simulink model "Control_sk_R3GDL"  (R2017b)
settings: Solver=ode45  StartTime=0.0  StopTime=12  MaxStep=1e-3  RelTol=1e-3  EnableMultiTasking=on
InitFcn:
  | Ts=1e-3;
StartFcn:
  | Ts=1e-3;
undefined symbols (not defined in the file or in its folder): CinematicaDirecta
settings Model: ExtModeTrigMode=oneshot  ExtModeArmWhenConnect=off  Creator=mortega  LastModifiedBy=Raúl
settings DataIOCC: SaveFormat=Array  SignalLoggingSaveFormat=ModelDataLogs
settings OptimizationCC: BlockReduction=off  BooleanDataType=off  ExpressionDepthLimit=2147483647  InitFltsAndDblsToZero=on  LifeSpan=inf
settings DebuggingCC: SaveWithParameterizedLinksMsg=none  UnderspecifiedInitializationDetection=Classic  MergeDetectMultiDrivingBlocksExec=none  SignalResolutionControl=TryResolveAllWithWarning  MultiTaskDSMMsg=warning  MultiTaskCondExecSysMsg=none  FcnCallInpInsideContextMsg=warning  StateNameClashWarn=warning  SFUnexpectedBacktrackingDiag=warning  SFNoUnconditionalDefaultTransitionDiag=warning  SFExecutionAtInitializationDiag=none
settings HardwareCC: ProdBitPerPointer=32  ProdBitPerSizeT=32  ProdBitPerPtrDiffT=32  ProdLargestAtomicFloat=None  ProdIntDivRoundTo=Undefined  ProdEndianess=Unspecified  ProdWordSize=32  ProdHWDeviceType=32-bit Generic  TargetUnknown=on
settings ModelReferenceCC: PropagateSignalLabelsOutOfModel=off
settings CodeAppCC: StateflowObjectComments=on
settings GRTTargetCC: TargetFcnLib=ansi_tfl_tmw.mat  TargetLangStandard=C89/C90 (ANSI)  GeneratePreprocessorConditionals=Disable all  CombineOutputUpdateFcns=off  GRTInterface=on
settings ConfigComp: CovMetricSettings=dw  CovHtmlReporting=on  CovSaveCumulativeToWorkspaceVar=on  CovSaveSingleToWorkspaceVar=on  CovExternalEMLEnable=off  CovSFcnEnable=off

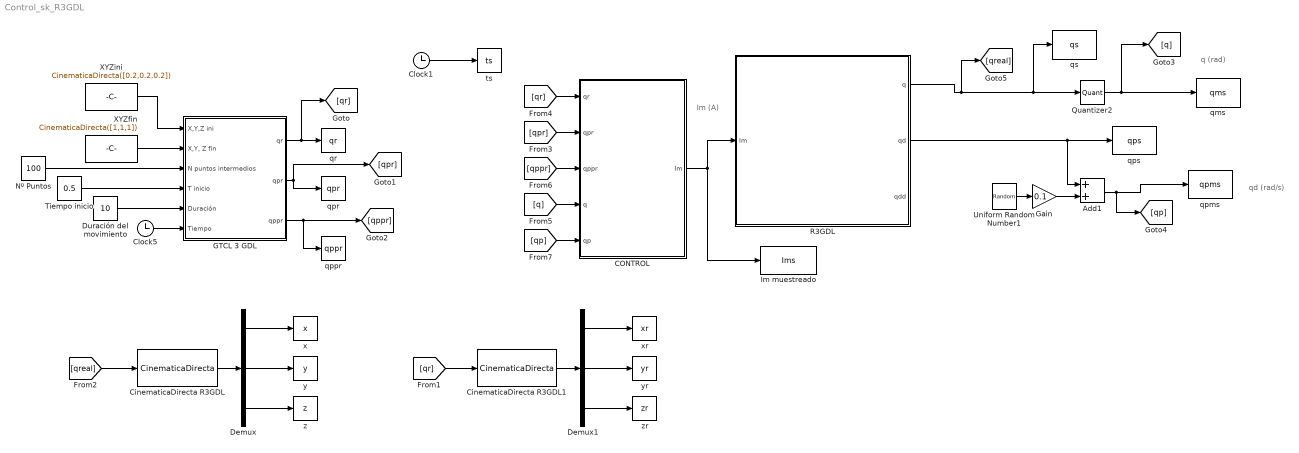
== system Control_sk_R3GDL ==
  note: q (rad)
  note: qd (rad/s)
  note: Im (A)
  Add1 : Sum
  CONTROL : Subsystem
  CinematicaDirecta R3GDL : MATLABFcn  MATLABFcn=CinematicaDirecta
  CinematicaDirecta R3GDL1 : MATLABFcn  MATLABFcn=CinematicaDirecta
  Clock1 : Clock
  Clock5 : Clock
  Demux : Demux  Outputs=3
  Demux1 : Demux  Outputs=3
  Duración del movimiento : Constant  Value=10
  GTCL 3 GDL : Subsystem
  Gain : Gain  Gain=0.1
  Im muestreado : ToWorkspace  VariableName=Ims  SampleTime=1e-3
  Nº Puntos : Constant  Value=100
  Quantizer2 : Quantizer  QuantizationInterval=2*pi/(512*25*100)
  R3GDL : Subsystem  mask(Control y Programación de Robots (4 GIERM)){NGrupo=3, q1_ini=0.2, q2_ini=0.2, q3_ini=0.2, Bl_q1=off, Bl_q2=off, Bl_q3=off, AccionamientoDirecto=on}
      mask prompts: NGrupo "Nº de GRUPO"; q1_ini "q1 inicial  (rad)"; q2_ini "q2 inicial (rad)"; q3_ini "q3_inicial (rad)"; Bl_q1 "Bloqueo q1"; Bl_q2 "Bloqueo q2"; Bl_q3 "Bloqueo q3"; AccionamientoDirecto "Accionamiento directo"
      mask help: Robot de 3 grados de libertad RRR
      mask Display:
      | image(imread('R3GDL_RRR.JPG'));
      | port_label('output', 1, 'q');
      | port_label('output', 2, 'qd');
      | port_label('output', 3, 'qdd');
      | port_label('input', 1, 'Im')
  Tiempo inicio : Constant  Value=0.5
  Uniform Random Number1 : UniformRandomNumber  Minimum=-157/1*0.02  Maximum=157/25*0.02  SampleTime=Ts
  XYZfin : Constant  Value=CinematicaDirecta([1,1,1])
  XYZini : Constant  Value=CinematicaDirecta([0.2,0.2,0.2])
  qms : ToWorkspace  VariableName=qms  SampleTime=Ts
  qpms : ToWorkspace  VariableName=qpms  SampleTime=Ts
  qppr : ToWorkspace  VariableName=qppr  SampleTime=Ts
  qpr : ToWorkspace  VariableName=qpr  SampleTime=Ts
  qps : ToWorkspace  VariableName=qps  SampleTime=Ts
  qr : ToWorkspace  VariableName=qr  SampleTime=Ts
  qs : ToWorkspace  VariableName=qs  SampleTime=Ts
  ts : ToWorkspace  VariableName=ts  SampleTime=Ts
  x : ToWorkspace  VariableName=x  SampleTime=Ts
  xr : ToWorkspace  VariableName=xr  SampleTime=Ts
  y : ToWorkspace  VariableName=y  SampleTime=Ts
  yr : ToWorkspace  VariableName=yr  SampleTime=Ts
  z : ToWorkspace  VariableName=z  SampleTime=Ts
  zr : ToWorkspace  VariableName=zr  SampleTime=Ts
  wires:
  Clock1/1 -> ts/1
  R3GDL/1(q) -> qs/1, Quantizer2/1, [qreal]
  Add1/1 -> [qp], qpms/1
  Uniform Random Number1/1 -> Gain/1
  R3GDL/2(qd) -> Add1/1, qps/1
  Clock5/1 -> GTCL 3 GDL/6(Tiempo)
  Duración del movimiento/1 -> GTCL 3 GDL/5(Duración)
  Tiempo inicio/1 -> GTCL 3 GDL/4(T inicio)
  Nº Puntos/1 -> GTCL 3 GDL/3(N puntos intermedios)
  XYZfin/1 -> GTCL 3 GDL/2("X,Y, Z fin")
  XYZini/1 -> GTCL 3 GDL/1(X,Y,Z ini)
  GTCL 3 GDL/1(qr) -> qr/1, [qr]
  GTCL 3 GDL/2(qpr) -> [qpr], qpr/1
  GTCL 3 GDL/3(qppr) -> qppr/1, [qppr]
  [qreal] -> CinematicaDirecta R3GDL/1
  CinematicaDirecta R3GDL/1 -> Demux/1
  Demux/1 -> x/1
  Demux/2 -> y/1
  Demux/3 -> z/1
  [qr] -> CinematicaDirecta R3GDL1/1
  CinematicaDirecta R3GDL1/1 -> Demux1/1
  Demux1/1 -> xr/1
  Demux1/2 -> yr/1
  Demux1/3 -> zr/1
  CONTROL/1(Im) -> R3GDL/1(Im), Im muestreado/1
  [qpr] -> CONTROL/2(qpr)
  [qr] -> CONTROL/1(qr)
  [q] -> CONTROL/4(q)
  [qppr] -> CONTROL/3(qppr)
  [qp] -> CONTROL/5(qp)
  Gain/1 -> Add1/2
  Quantizer2/1 -> [q], qms/1

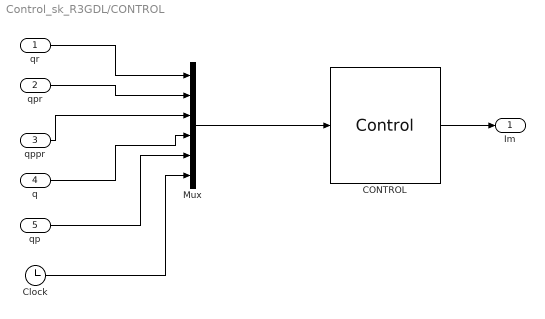
== system Control_sk_R3GDL/CONTROL ==
  qr : Inport
  qpr : Inport  Port=2
  qppr : Inport  Port=3
  q : Inport  Port=4
  qp : Inport  Port=5
  CONTROL : MATLABFcn  MATLABFcn=Control  OutputDimensions=3  SampleTime=0.001
  Clock : Clock
  Mux : Mux  Inputs=6
  Im : Outport
  wires:
  Mux/1 -> CONTROL/1
  CONTROL/1 -> Im/1
  qr/1 -> Mux/1
  qpr/1 -> Mux/2
  qppr/1 -> Mux/3
  q/1 -> Mux/4
  qp/1 -> Mux/5
  Clock/1 -> Mux/6

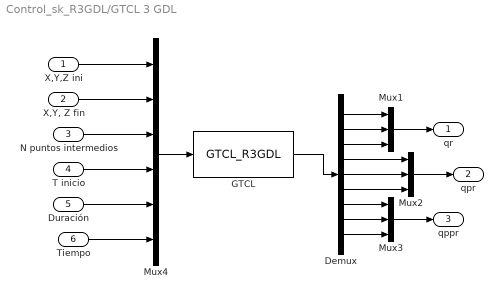
== system Control_sk_R3GDL/GTCL 3 GDL ==
  X,Y,Z ini : Inport
  "X,Y, Z fin" : Inport  Port=2
  N puntos intermedios : Inport  Port=3
  T inicio : Inport  Port=4
  Duración : Inport  Port=5
  Tiempo : Inport  Port=6
  Demux : Demux  Outputs=9
  GTCL : MATLABFcn  MATLABFcn=GTCL_R3GDL  OutputDimensions=9  SampleTime=10*0.001
  Mux1 : Mux  Inputs=3
  Mux2 : Mux  Inputs=3
  Mux3 : Mux  Inputs=3
  Mux4 : Mux  Inputs=6
  qr : Outport
  qpr : Outport  Port=2
  qppr : Outport  Port=3
  wires:
  Mux1/1 -> qr/1
  Mux4/1 -> GTCL/1
  X,Y,Z ini/1 -> Mux4/1
  "X,Y, Z fin"/1 -> Mux4/2
  N puntos intermedios/1 -> Mux4/3
  T inicio/1 -> Mux4/4
  Duración/1 -> Mux4/5
  Tiempo/1 -> Mux4/6
  GTCL/1 -> Demux/1
  Demux/1 -> Mux1/1
  Demux/2 -> Mux1/2
  Demux/3 -> Mux1/3
  Mux2/1 -> qpr/1
  Demux/4 -> Mux2/1
  Demux/5 -> Mux2/2
  Demux/6 -> Mux2/3
  Mux3/1 -> qppr/1
  Demux/7 -> Mux3/1
  Demux/8 -> Mux3/2
  Demux/9 -> Mux3/3

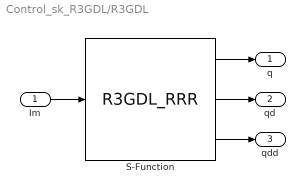
== system Control_sk_R3GDL/R3GDL ==
  Im : Inport
  S-Function : S-Function  FunctionName=R3GDL_RRR  Parameters=[q1_ini; q2_ini; q3_ini]; [Bl_q1; Bl_q2; Bl_q3]; AccionamientoDirecto; NGrupo  SFunctionDeploymentMode=off  EnableBusSupport=off
  q : Outport
  qd : Outport  Port=2
  qdd : Outport  Port=3
  wires:
  Im/1 -> S-Function/1
  S-Function/1 -> q/1
  S-Function/2 -> qd/1
  S-Function/3 -> qdd/1
